simulink subsystem "Strecke"  (R2021b)
settings: Solver=VariableStepAuto  StartTime=0.0  StopTime=10.0  RelTol=1e-3
values from neighbouring files (symbols this model uses):
  DriftGain = 1    [RaketeParameter.m]
  FlapGain = 1.3178    [RaketeParameter.m]    (also in SimulationParameter.m = 0.00716)
  Gravitation = 9.8067    [RaketeParameter.m]    (also in SimulationParameter.m)
  PitchTraegheit = 0.0362    [RaketeParameter.m]    (also in SimulationParameter.m = 0.0424436)
  PropGain = (ObjectMass*Gravitation)/0.8    [RaketeParameter.m]    (also in SimulationParameter.m = -(ObjectMass*Gravitation)/0.8)
  PropOffset = 0.08    [RaketeParameter.m]    (also in SimulationParameter.m = 0.09)
  RollTraegheit = 0.0430    (= 0.043)    [RaketeParameter.m]    (also in SimulationParameter.m = 0.0459025)
  YawTraegheit = 0.0335    [RaketeParameter.m]    (also in SimulationParameter.m = 0.0360284)
undefined symbols (not defined in the file or in its folder): ObjectMass
settings Model: Creator=tim  LastModifiedBy=tim

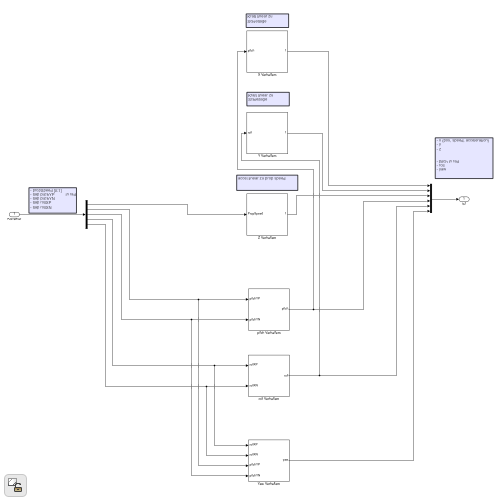
[thumbnail: Simulink's stored preview of the top-level diagram]
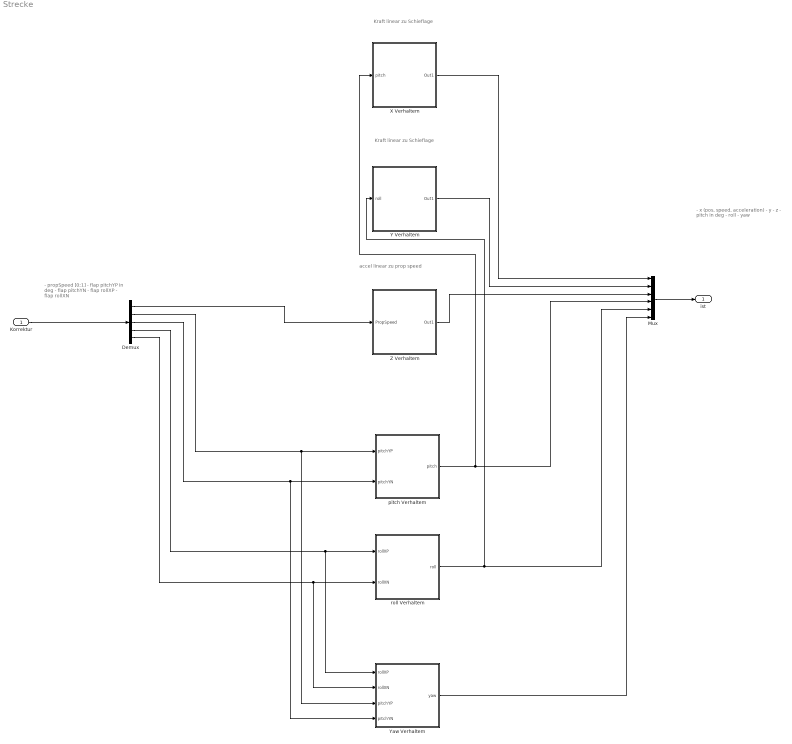
== system Strecke ==
  note: Kraft linear zu
      | Schieflage
  note: accel linear zu prop speed
  note: - propSpeed [0;1]
      | - flap pitchYP          in deg
      | - flap pitchYN
      | - flap rollXP
      | - flap rollXN
  note: - x (pos, speed, acceleration)
      | - y
      | - z
      |
      |
      | - pitch in deg
      | - roll
      | - yaw
  note: Kraft linear zu
      | Schieflage
  Korrektur : Inport
  Demux : Demux  Outputs=5
  Mux : Mux  Inputs=6
  X Verhaltem : Subsystem
  Y Verhaltem : Subsystem
  Yaw Verhaltem : Subsystem
  Z Verhaltem : Subsystem
  pitch Verhaltem : Subsystem
  roll Verhaltem : Subsystem
  ist : Outport
  wires:
  Demux/1 -> Z Verhaltem/1(PropSpeed)
  Mux/1 -> ist/1
  Z Verhaltem/1(Out1) -> Mux/3
  Korrektur/1 -> Demux/1
  X Verhaltem/1(Out1) -> Mux/1
  Y Verhaltem/1(Out1) -> Mux/2
  Demux/2 -> pitch Verhaltem/1(pitchYP), Yaw Verhaltem/3(pitchYP)
  Demux/3 -> pitch Verhaltem/2(pitchYN), Yaw Verhaltem/4(pitchYN)
  Demux/4 -> Yaw Verhaltem/1(rollXP), roll Verhaltem/1(rollXP)
  Demux/5 -> roll Verhaltem/2(rollXN), Yaw Verhaltem/2(rollXN)
  roll Verhaltem/1(roll) -> Mux/5, Y Verhaltem/1(roll)
  Yaw Verhaltem/1(yaw) -> Mux/6
  pitch Verhaltem/1(pitch) -> Mux/4, X Verhaltem/1(pitch)

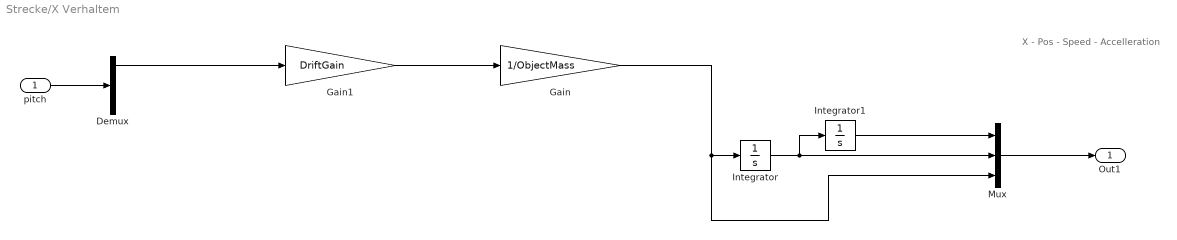
== system Strecke/X Verhaltem ==
  note: X
      | - Pos
      | - Speed
      | - Accelleration
  pitch : Inport
  Demux : Demux  Outputs=3
  Gain : Gain  Gain=1/ObjectMass
  Gain1 : Gain  Gain=DriftGain
  Integrator : Integrator
  Integrator1 : Integrator
  Mux : Mux  Inputs=3
  Out1 : Outport
  wires:
  Gain1/1 -> Gain/1
  Gain/1 -> Integrator/1, Mux/3
  Integrator1/1 -> Mux/1
  Integrator/1 -> Mux/2, Integrator1/1
  Demux/1 -> Gain1/1
  pitch/1 -> Demux/1
  Mux/1 -> Out1/1

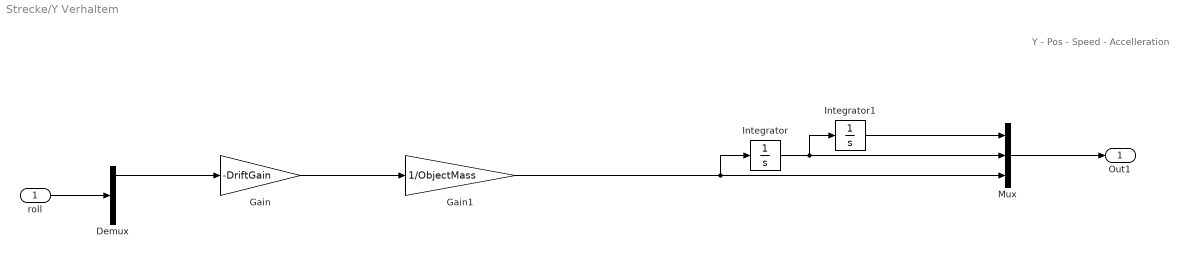
== system Strecke/Y Verhaltem ==
  note: Y
      | - Pos
      | - Speed
      | - Accelleration
  roll : Inport
  Demux : Demux  Outputs=3
  Gain : Gain  Gain=-DriftGain
  Gain1 : Gain  Gain=1/ObjectMass
  Integrator : Integrator
  Integrator1 : Integrator
  Mux : Mux  Inputs=3
  Out1 : Outport
  wires:
  Gain1/1 -> Mux/3, Integrator/1
  Gain/1 -> Gain1/1
  Demux/1 -> Gain/1
  Integrator1/1 -> Mux/1
  Integrator/1 -> Mux/2, Integrator1/1
  roll/1 -> Demux/1
  Mux/1 -> Out1/1

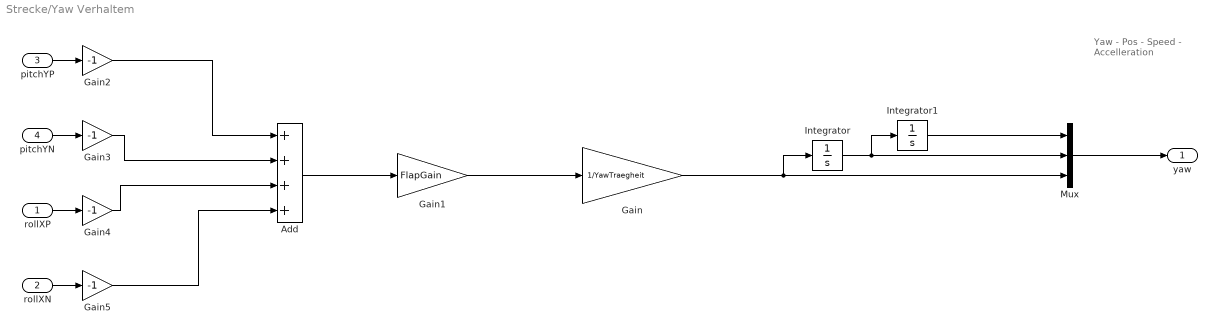
== system Strecke/Yaw Verhaltem ==
  note: Yaw
      | - Pos
      | - Speed
      | - Accelleration
  rollXP : Inport
  rollXN : Inport  Port=2
  pitchYP : Inport  Port=3
  pitchYN : Inport  Port=4
  Add : Sum  Inputs=++++
  Gain : Gain  Gain=1/YawTraegheit
  Gain1 : Gain  Gain=FlapGain
  Gain{2..5} (4 alike) : Gain  Gain=-1
  Integrator : Integrator
  Integrator1 : Integrator
  Mux : Mux  Inputs=3
  yaw : Outport
  wires:
  Mux/1 -> yaw/1
  Gain5/1 -> Add/4
  Gain4/1 -> Add/3
  Gain3/1 -> Add/2
  Gain2/1 -> Add/1
  Gain/1 -> Mux/3, Integrator/1
  Add/1 -> Gain1/1
  rollXN/1 -> Gain5/1
  rollXP/1 -> Gain4/1
  Gain1/1 -> Gain/1
  pitchYN/1 -> Gain3/1
  pitchYP/1 -> Gain2/1
  Integrator1/1 -> Mux/1
  Integrator/1 -> Mux/2, Integrator1/1

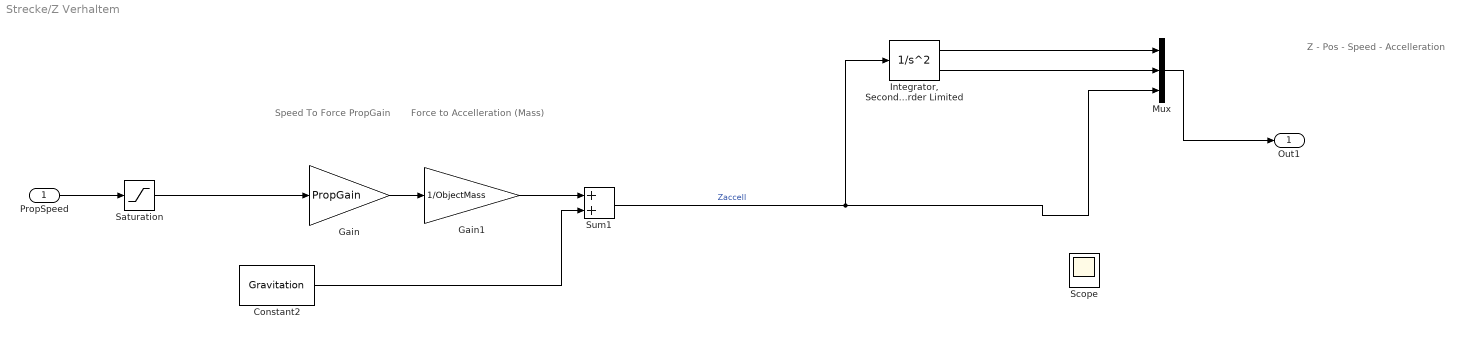
== system Strecke/Z Verhaltem ==
  note: Force to Accelleration
      | (Mass)
  note: Z
      | - Pos
      | - Speed
      | - Accelleration
  note: Speed To Force
      | PropGain
  PropSpeed : Inport
  Constant2 : Constant  Value=Gravitation
  Gain : Gain  Gain=PropGain
  Gain1 : Gain  Gain=1/ObjectMass
  "Integrator, Second-Order Limited" : SecondOrderIntegrator  LimitX=on  UpperLimitX=0  LowerLimitX=-1000000  LimitDXDT=on
  Mux : Mux  Inputs=3
  Saturation : Saturate  UpperLimit=0  LowerLimit=-1
  Scope : Scope  NumInputPorts=3
  Sum1 : Sum
  Out1 : Outport
  wires:
  Saturation/1 -> Gain/1
  Gain1/1 -> Sum1/1
  "Integrator, Second-Order Limited"/2 -> Mux/2
  "Integrator, Second-Order Limited"/1 -> Mux/1
  Sum1/1 -> Mux/3, "Integrator, Second-Order Limited"/1  "Zaccell"
  Gain/1 -> Gain1/1
  Constant2/1 -> Sum1/2
  PropSpeed/1 -> Saturation/1
  Mux/1 -> Out1/1

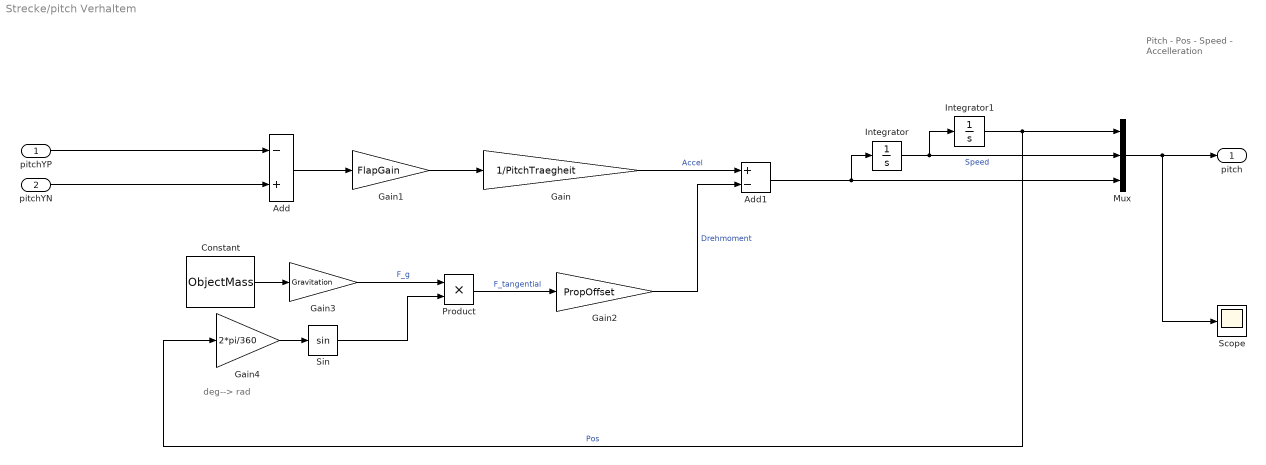
== system Strecke/pitch Verhaltem ==
  note: Pitch
      | - Pos
      | - Speed
      | - Accelleration
  note: deg--> rad
  pitchYP : Inport
  pitchYN : Inport  Port=2
  Add : Sum  Inputs=-+
  Add1 : Sum  Inputs=+-
  Constant : Constant  Value=ObjectMass
  Gain : Gain  Gain=1/PitchTraegheit
  Gain1 : Gain  Gain=FlapGain
  Gain2 : Gain  Gain=PropOffset
  Gain3 : Gain  Gain=Gravitation
  Gain4 : Gain  Gain=2*pi/360
  Integrator : Integrator
  Integrator1 : Integrator
  Mux : Mux  Inputs=3
  Product : Product
  Scope : Scope
  Sin : Trigonometry
  pitch : Outport
  wires:
  Gain4/1 -> Sin/1
  Product/1 -> Gain2/1  "F_tangential"
  Sin/1 -> Product/2
  Gain3/1 -> Product/1  "F_g"
  Constant/1 -> Gain3/1
  Gain2/1 -> Add1/2  "Drehmoment"
  Gain/1 -> Add1/1  "Accel"
  Add1/1 -> Mux/3, Integrator/1
  Add/1 -> Gain1/1
  pitchYN/1 -> Add/2
  Gain1/1 -> Gain/1
  Integrator1/1 -> Mux/1, Gain4/1  "Pos"
  Integrator/1 -> Mux/2, Integrator1/1  "Speed"
  pitchYP/1 -> Add/1
  Mux/1 -> Scope/1, pitch/1

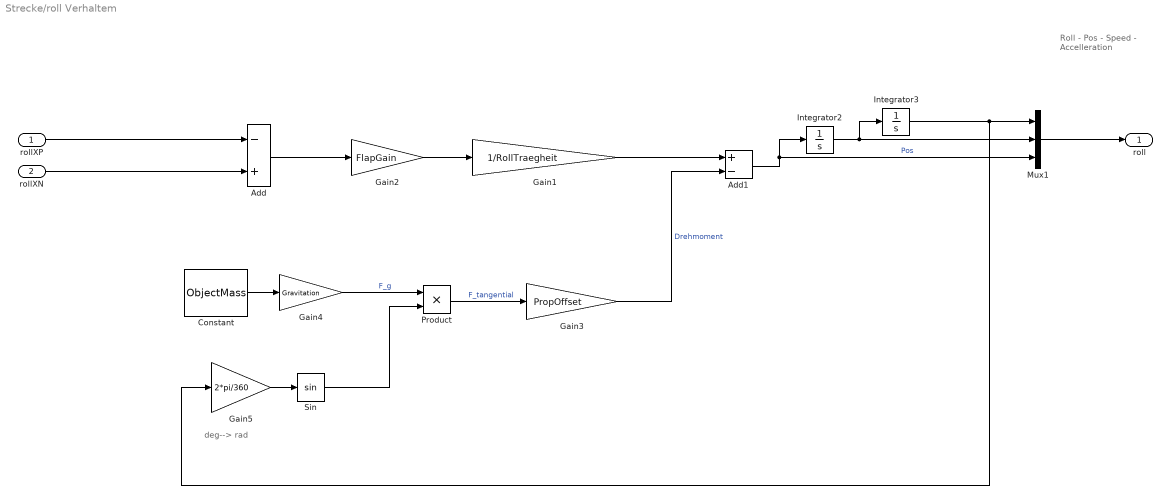
== system Strecke/roll Verhaltem ==
  note: deg--> rad
  note: Roll
      | - Pos
      | - Speed
      | - Accelleration
  rollXP : Inport
  rollXN : Inport  Port=2
  Add : Sum  Inputs=-+
  Add1 : Sum  Inputs=+-
  Constant : Constant  Value=ObjectMass
  Gain1 : Gain  Gain=1/RollTraegheit
  Gain2 : Gain  Gain=FlapGain
  Gain3 : Gain  Gain=PropOffset
  Gain4 : Gain  Gain=Gravitation
  Gain5 : Gain  Gain=2*pi/360
  Integrator2 : Integrator
  Integrator3 : Integrator
  Mux1 : Mux  Inputs=3
  Product : Product
  Sin : Trigonometry
  roll : Outport
  wires:
  Gain5/1 -> Sin/1
  Integrator2/1 -> Mux1/2, Integrator3/1
  Gain1/1 -> Add1/1
  Gain4/1 -> Product/1  "F_g"
  Sin/1 -> Product/2
  Add1/1 -> Integrator2/1, Mux1/3  "Pos"
  Gain3/1 -> Add1/2  "Drehmoment"
  Constant/1 -> Gain4/1
  Product/1 -> Gain3/1  "F_tangential"
  rollXP/1 -> Add/1
  Add/1 -> Gain2/1
  Gain2/1 -> Gain1/1
  Mux1/1 -> roll/1
  rollXN/1 -> Add/2
  Integrator3/1 -> Mux1/1, Gain5/1
